simulink model "find6DOFSnellMin_th"  (R2018b)
settings: Solver=ode8  StartTime=0.0  StopTime=index - 1  FixedStep=0.2  RelTol=1e-3  EnableMultiTasking=on
values from neighbouring files (symbols this model uses):
  botDot = timeseries(botDot)    [find6DOFSnellMin_ts.m]
  sideDot = timeseries(sideDot)    [find6DOFSnellMin_ts.m]
  slntDot = timeseries(slntDot)    [find6DOFSnellMin_ts.m]
libraries: find6DOFSnellMin_cl x1
settings Model: SimulationMode=external  Creator=MAE-NCSUCORE  LastModifiedBy=MAE-NCSUCORE
settings SolverCC: ConcurrentTasks=on  AutoInsertRateTranBlk=on
settings DataIOCC: SaveFormat=StructureWithTime
settings OptimizationCC: BlockReduction=off  OptimizeBlockIOStorage=off  BufferReuse=off  GlobalBufferReuse=off  ExpressionFolding=off  LocalBlockOutputs=off  OptimizeDataStoreBuffers=off  BusAssignmentInplaceUpdate=off
settings HardwareCC: ProdBitPerPointer=32  ProdBitPerSizeT=32  ProdBitPerPtrDiffT=32  ProdLargestAtomicFloat=None  ProdWordSize=32  ProdLongLongMode=on  ProdHWDeviceType=Generic->32-bit x86 compatible
settings RTWCC: SystemTargetFile=slrt.tlc  TemplateMakefile=slrt_default_tmf  Description=Simulink Real-Time  CodeExecutionProfiling=on  RTWCompilerOptimization=on
settings SimulinkRealTimeCC: SupportVariableSizeSignals=on  PreserveStateflowLocalDataDimensions=off  RL32ObjectName=tg2  xPCisDefaultEnv=off  xPCTargetPCEnvName=Machine2  xPCConcurrentTasks=on

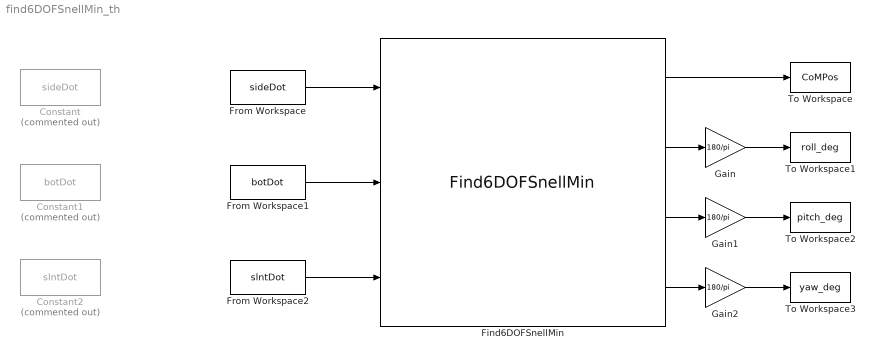
== system find6DOFSnellMin_th ==
  Constant : Constant  Commented=on  Value=sideDot
  Constant1 : Constant  Commented=on  Value=botDot
  Constant2 : Constant  Commented=on  Value=slntDot
  Find6DOFSnellMin : find6DOFSnellMin_cl/Find6DOFSnellMin  imageDims_px=params.sideImageSize_px.Value  initialCoMPositionVec_cm=params.initCoMPosVec_cm.Value  initialEulerAngles_deg=params.initEulerAng_deg.Value  indxOfRefVec=params.indexOfRefractionA.Value  glassThickness_cm=params.glassThickness_cm.Value  cameraFOVAngles_deg=params.cameraFOV_deg.Value  sideEulerAngles_deg=params.sideCamEulAng_deg.Value  sideCamPositionVec_cm=params.sideCamPosVec_cm.Value  sideCamDistToGlass_cm=params.sideDistancetoGlass_cm.Value  botEulerAngles_deg=params.botCamEulAng_deg.Value  botCamPositionVec_cm=params.botCamPosVec_cm.Value  botCamDistToGlass_cm=params.botDistancetoGlass_cm.Value  slantEulerAngles_deg=params.slntCamEulAng_deg.Value  slantCamPositionVec_cm=params.slntCamPosVec_cm.Value  slantCamDistToGlass_cm=params.slntDistancetoGlass_cm.Value  sideSeparation_cm=params.sideDotSepDist_cm.Value  sidePositionVecBF_cm=params.sideDotPosVec_cm.Value  bottomASeparation_cm=params.botADotSepDist_cm.Value  botAPositionVecBF_cm=params.botADotPosVec_cm.Value  bottomBSeparation_cm=params.botBDotSepDist_cm.Value  botBPositionVecBF_cm=params.botBDotPosVec_cm.Value
  From Workspace : FromWorkspace  VariableName=sideDot  SampleTime=0
  From Workspace1 : FromWorkspace  VariableName=botDot  SampleTime=0
  From Workspace2 : FromWorkspace  VariableName=slntDot  SampleTime=0
  Gain : Gain  Gain=180/pi
  Gain1 : Gain  Gain=180/pi
  Gain2 : Gain  Gain=180/pi
  To Workspace : ToWorkspace  VariableName=CoMPos  SaveFormat=Timeseries  SampleTime=-1
  To Workspace1 : ToWorkspace  VariableName=roll_deg  SaveFormat=Timeseries  SampleTime=-1
  To Workspace2 : ToWorkspace  VariableName=pitch_deg  SaveFormat=Timeseries  SampleTime=-1
  To Workspace3 : ToWorkspace  VariableName=yaw_deg  SaveFormat=Timeseries  SampleTime=-1
  wires:
  Find6DOFSnellMin/1 -> To Workspace/1
  Find6DOFSnellMin/2 -> Gain/1
  Gain/1 -> To Workspace1/1
  Find6DOFSnellMin/4 -> Gain2/1
  Find6DOFSnellMin/3 -> Gain1/1
  Gain1/1 -> To Workspace2/1
  Gain2/1 -> To Workspace3/1
  From Workspace/1 -> Find6DOFSnellMin/1
  From Workspace1/1 -> Find6DOFSnellMin/2
  From Workspace2/1 -> Find6DOFSnellMin/3
